simulink model "q910"  (Simulink 8.3)
settings: Solver=ode45  StartTime=0.0  StopTime=100  RelTol=1e-3
values from neighbouring files (symbols this model uses):
  a = a0+delta_a    (= 3.4)    [q315.m]    (also in q315b_m.m)
  K = P * phi(:,i)* inv(lambda + phi(:,i)'* P * phi(:,i))    [ex310.m]    (also in ex378.m; ex39.m; q311.m; q315.m)
  Ki = 1.5    [q315.m]    (also in q315b_m.m)
libraries: simulink x1
settings Model: Creator=Nelson  LastModifiedBy=erobotica
settings DataIOCC: SignalLoggingSaveFormat=Dataset
settings GRTTargetCC: CombineOutputUpdateFcns=on  GRTInterface=off

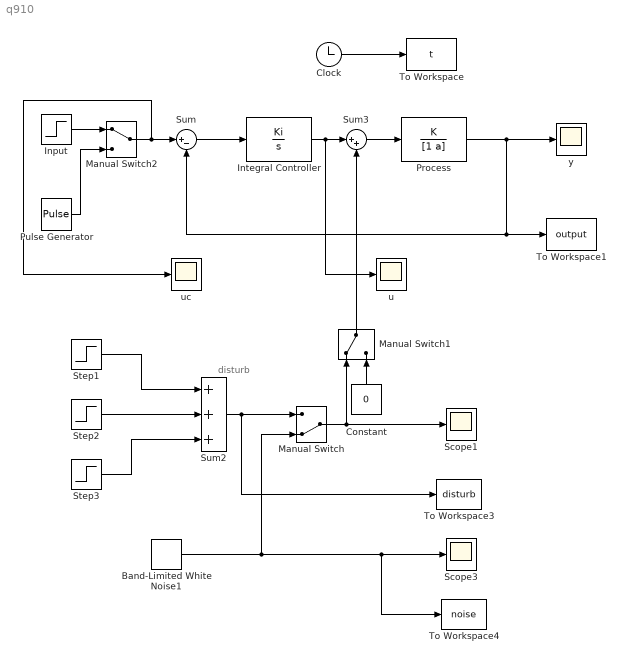
== system q910 ==
  note: disturb
  Band-Limited White Noise1 : simulink/Sources/Band-Limited White Noise  Cov=[0.01]  Ts=0.01  seed=[23341]
  Clock : Clock
  Constant : Constant  Value=0
  "Input " : Step  Time=0  SampleTime=0
  Integral Controller : TransferFcn  Numerator=Ki  Denominator=[1 0]
  Manual Switch : ManualSwitch  CurrentSetting=0
  Manual Switch1 : ManualSwitch
  Manual Switch2 : ManualSwitch
  Process : TransferFcn  Numerator=K  Denominator=[1 a]
  Pulse Generator : DiscretePulseGenerator  PulseType=Time based  Period=50  PulseWidth=50
  Scope1 : Scope
      settings: SaveName=ScopeData2
  Scope3 : Scope
      settings: SaveName=ScopeData3
  Step1 : Step  Time=0  After=-1  SampleTime=0
  Step2 : Step  Time=6  After=3  SampleTime=0
  Step3 : Step  Time=15  After=-1  SampleTime=0
  Sum : Sum  Inputs=|+-
  Sum2 : Sum  Inputs=+++
  Sum3 : Sum  Inputs=|++
  To Workspace : ToWorkspace  VariableName=t  SampleTime=-1
  To Workspace1 : ToWorkspace  VariableName=output  SampleTime=-1
  To Workspace3 : ToWorkspace  VariableName=disturb  SampleTime=-1
  To Workspace4 : ToWorkspace  VariableName=noise  SampleTime=-1
  u : Scope
      settings: SaveName=u  MaxDataPoints=500000
  uc : Scope
      settings: SaveName=uc  MaxDataPoints=500000
  y : Scope
      settings: SaveName=y  MaxDataPoints=500000
  wires:
  Process/1 -> Sum/2, To Workspace1/1, y/1
  Sum/1 -> Integral Controller/1
  Clock/1 -> To Workspace/1
  Step2/1 -> Sum2/2
  Step1/1 -> Sum2/1
  Step3/1 -> Sum2/3
  Sum2/1 -> Manual Switch/1, To Workspace3/1
  Manual Switch/1 -> Manual Switch1/1, Scope1/1
  Band-Limited White Noise1/1 -> Manual Switch/2, Scope3/1, To Workspace4/1
  Integral Controller/1 -> u/1, Sum3/1
  Sum3/1 -> Process/1
  Manual Switch1/1 -> Sum3/2
  Constant/1 -> Manual Switch1/2
  "Input "/1 -> Manual Switch2/1
  Manual Switch2/1 -> uc/1, Sum/1
  Pulse Generator/1 -> Manual Switch2/2
